simulink model "motor_bearing_fault"  (R2025a)
settings: Solver=FixedStepAuto  StartTime=0  StopTime=5  FixedStep=1e-4  RelTol=1e-3
undefined symbols (not defined in the file): f_supply, fault_severity, Torque_in, V_in
libraries: spsAsynchronousMachineSIUnitsLib x1, spsThreePhaseSourceLib x1, spspowerguiLib x1
settings Model: Creator=User  LastModifiedBy=User
settings DataIOCC: SaveOutput=off  DSMLogging=off  ReturnWorkspaceOutputs=off

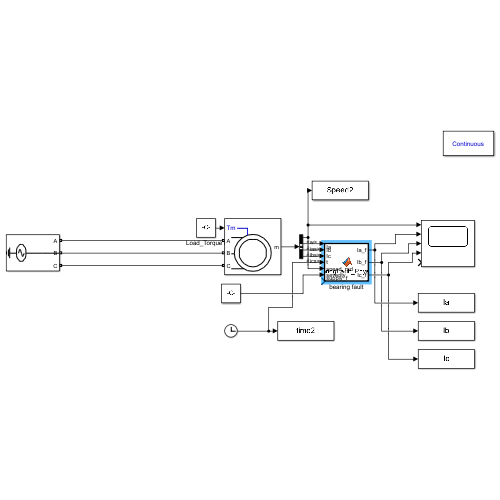
[thumbnail: Simulink's stored preview of the top-level diagram]
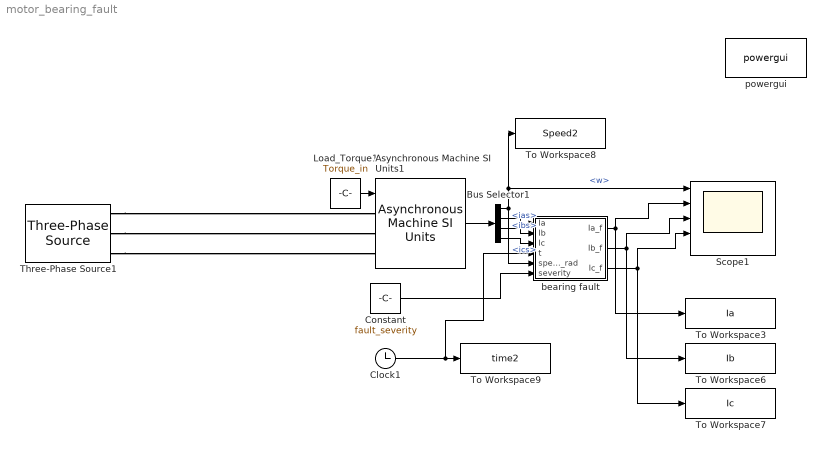
== system motor_bearing_fault ==
  Asynchronous Machine SI Units1 : spsAsynchronousMachineSIUnitsLib/Asynchronous Machine SI Units  RotorType=Squirrel-cage  PresetModel=No  MechanicalLoad=Torque Tm  ShowDetailedParameters=on  ReferenceFrame=Stationary  Units=SI  MeasurementBus=on  NominalParameters=[7500 400 50]  VoltageRatio=1  Stator=[1.405 0.005839]  Rotor=[1.395 0.005839]  Cage1=[0.4155 0.002066]  Cage2=[0.4168 0.0003495]  Lm=0.1722  Mechanical=[0.0131 0.001 2]  PolePairs=2  InitialConditions=[0 0 0 0 0 0 0 0]  SimulateSaturation=off  Saturation=[14.03593122, 27.81365428, 53.79336849, 72.68890987, 97.98006896, 148.6815601, 215.7428561, 302.9841135, 428.7778367 ; 230, 322, 414, 460, 506, 552, 598, 644, 690]  LoadFlowParameters=1492000  TsPowergui=0  TsBlock=-1  IterativeModel=Trapezoidal non iterative  IterativeDiscreteModel=Trapezoidal non iterative  Pmec=1.492e+006
  Bus Selector1 : BusSelector  OutputSignals=w,ias,ibs,ics
  Clock1 : Clock
  Constant : Constant  Value=fault_severity
  Load_Torque1 : Constant  Value=Torque_in
  Scope1 : Scope  NumInputPorts=5
      settings: ActiveDisplayYMinimum=-0.049617664684487431  ActiveDisplayYMaximum=0.049617664684487604
  Three-Phase Source1 : spsThreePhaseSourceLib/Three-Phase Source  InternalConnection=Yg  VoltagePhases=on  Voltage=400  PhaseAngle=0  Voltage_phases=[V_in V_in V_in]/sqrt(3)  PhaseAngles_phases=[0 -120 +120]  Frequency=f_supply  NonIdealSource=off  SpecifyImpedance=off  Resistance=0.8929  Inductance=16.58e-3  ShortCircuitLevel=100e6  BaseVoltage=25e3  XRratio=7  BusType=swing  Pref=10e3  Qref=0  Prefabc=[10e3, 10e3, 10e3]  Qrefabc=[0, 0, 0]  Qmin=-inf  Qmax=inf
  To Workspace3 : ToWorkspace  VariableName=Ia  SampleTime=-1
  To Workspace6 : ToWorkspace  VariableName=Ib  SampleTime=-1
  To Workspace7 : ToWorkspace  VariableName=Ic  SampleTime=-1
  To Workspace8 : ToWorkspace  VariableName=Speed2  SampleTime=-1
  To Workspace9 : ToWorkspace  VariableName=time2  SampleTime=-1
  bearing fault : MATLAB Function  TreatAsAtomicUnit=on
  powergui : spspowerguiLib/powergui  Priority=1  SimulationMode=Continuous  SampleTime=50e-6  frequency=60  Iterations=50  frequencyindice=50  Pbase=100e6  ErrMax=1e-4  UnitsV=kV  UnitsW=MW  buscounter=0  FunctionMessages=off  echomessages=off  EnableUseOfTLC=off  CurrentSourceSwitches=off  DisableSnubberDevices=off  DisableRonSwitches=off  DisableVfSwitches=off  DisplayEquations=off  AutomaticDiscreteSolvers=off  SolverType=Tustin/Backward Euler (TBE)  Interpol=off  ExternalGateDelay=off  methode=off  Ts=100  x0status=blocks  SPID=on  SwTol=0  HookPort=off  NonlinearTolerance=1e-4  nMaxIteration=100  ContinueOnMaxIteration=off  RestoreLinks=warning  ResistiveCurrentMeasurement=off  Frange=[0:2:500]  Ylog=off  Xlog=on  ShowGrid=off  save=off  variable=ZData  structure=0  ZoomFFT=off  StartTime=0.0  cycles=1  DisplayStyle=1  fundamental=60  FreqAxis=off  MaxFrequency=1000  frequencyindicesteady=1  RmsSteady=1  display=off
  wires:
  Load_Torque1/1 -> Asynchronous Machine SI Units1/1
  Bus Selector1/1 -> To Workspace8/1, Scope1/1, bearing fault/5(speed_rad)  "<w>"
  Asynchronous Machine SI Units1/1 -> Bus Selector1/1
  Clock1/1 -> bearing fault/4(t), To Workspace9/1
  bearing fault/3(Ic_f) -> Scope1/4, To Workspace7/1
  bearing fault/1(Ia_f) -> Scope1/2, To Workspace3/1
  bearing fault/2(Ib_f) -> Scope1/3, To Workspace6/1
  Bus Selector1/2 -> bearing fault/1(Ia)  "<ias>"
  Bus Selector1/3 -> bearing fault/2(Ib)  "<ibs>"
  Bus Selector1/4 -> bearing fault/3(Ic)  "<ics>"
  Constant/1 -> bearing fault/6(severity)
  connections:
  Three-Phase Source1/RConn3 -- Asynchronous Machine SI Units1/LConn3
  Three-Phase Source1/RConn1 -- Asynchronous Machine SI Units1/LConn1
  Three-Phase Source1/RConn2 -- Asynchronous Machine SI Units1/LConn2

== matlab function motor_bearing_fault/bearing fault ==
  data: Ia input; Ia_f output; Ib input; Ic input; t input; Ib_f output; Ic_f output; speed_rad input; severity input
function [Ia_f, Ib_f, Ic_f] = BearingFault_Physical( ...
    Ia, Ib, Ic, t, speed_rad, severity)
%#codegen
% PHYSICAL BEARING FAULT MODEL for Induction Motor
%
% fault_type:
%   1 = Outer race fault
%   2 = Inner race fault
%   3 = Ball fault
%   4 = General bearing roughness
%
% Example usage:
% [Ia_f,Ib_f,Ic_f] = BearingFault_Physical(Ia,Ib,Ic,t,1500,1);
    rpm = speed_rad * 9.549;
    % Motor + Bearing constants
    mech_f = rpm/60;                      % mechanical freq

    % Bearing geometry (Example 6305)
    nb = 8;                               % number of rolling balls
    Bd = 8.5e-3;                           % ball diameter (m)
    Pd = 39e-3;                            % pitch diameter (m)
    contact = 0;                           % contact angle (rad)
    
    % Calculate fault signature frequencies
    BPFO = (nb/2)*(1 - Bd/Pd*cos(contact)) * mech_f;         % Outer race

    ff = BPFO;

    % -----------------------------------------------------------
    % 1) HIGH-FREQUENCY VIBRATION MODULATION (bearing vibration)
    % -----------------------------------------------------------
    hf_modulation = severity * 0.2 * sin(2*pi*ff*t) + ...
                    severity * 0.1 * sin(2*pi*2*ff*t);

    % -----------------------------------------------------------
    % 2) IMPULSE TRAIN (bearing rolling element hits)
    % -----------------------------------------------------------
    impulse_train = zeros(size(t));
    hit_period = 1/ff;  
    for k = 1:length(t)
        % impulses at bearing fault frequency
        if mod(t(k), hit_period) < 0.0004
            impulse_train(k) = severity * 0.5 * exp(-800*(mod(t(k),hit_period)));
        end
    end

    % -----------------------------------------------------------
    % 3) CURRENT MODULATION (bearing load variation)
    % -----------------------------------------------------------
    % load torque ripple → current ripple
    current_modulation = severity * 0.3 * sin(2*pi*ff*t);

    % -----------------------------------------------------------
    % Combine all effects into a single bearing fault signal
    % -----------------------------------------------------------
    fault_signal = hf_modulation + impulse_train + current_modulation;

    % -----------------------------------------------------------
    % 4) APPLY TO PHASE CURRENTS WITH PROPER UNBALANCE
    % -----------------------------------------------------------
    % bearing faults produce mechanical vibration → uneven air gap →
    % slight unbalance in line currents.
    Ia_f = Ia + fault_signal;
    Ib_f = Ib + 0.7 * fault_signal .* cos(2*pi/3);
    Ic_f = Ic + 0.7 * fault_signal .* cos(4*pi/3);

end
